simulink library "downlink_labels_lib"  (Simulink 6.6)
libraries: Telemetry_Lib x4, simulink x1
settings Model: Creator=cbuttril  LastModifiedBy=cbuttril

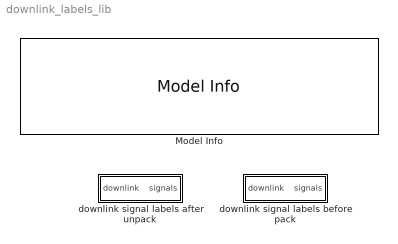
== system downlink_labels_lib ==
  Model Info : simulink/Model-Wide Utilities/Model Info  SystemSampleTime=-1  InitialBlockCM=None  BlockCM=None  Frame=on  DisplayStringWithTags=|  HorizontalTextAlignment=Center  LeftAlignmentValue=0.5  SourceBlockDiagram=downlink_labels_lib  TagMaxNumber=20
      | Developed using Matlab Release 2007a
      | 
      | SVN:%<ModelVersion>
      | Last modifed by %<LastModifiedBy> on %<LastModificationDate>
  downlink signal labels after unpack : Subsystem
  downlink signal labels before pack : Subsystem

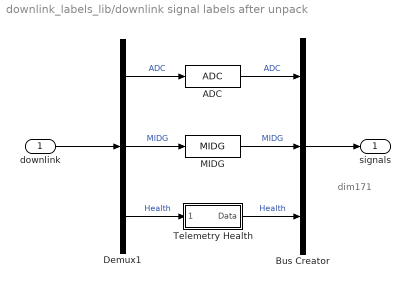
== system downlink_labels_lib/downlink signal labels after unpack ==
  note: dim171
  downlink : Inport
  ADC : Telemetry_Lib/ADC  SystemSampleTime=-1
  Bus Creator : BusCreator  Inputs=3
  Demux1 : Demux  Outputs=[62 99 10]
  MIDG : Telemetry_Lib/MIDG  SystemSampleTime=-1
  Telemetry Health : Subsystem
  signals : Outport  PortDimensions=171
  wires:
  Bus Creator/1 -> signals/1
  ADC/1 -> Bus Creator/1  "ADC"
  Demux1/1 -> ADC/1  "ADC"
  Telemetry Health/1(Data) -> Bus Creator/3  "Health"
  MIDG/1 -> Bus Creator/2  "MIDG"
  Demux1/3 -> Telemetry Health/1(Health)  "Health"
  Demux1/2 -> MIDG/1  "MIDG"
  downlink/1 -> Demux1/1

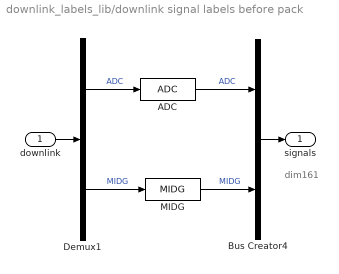
== system downlink_labels_lib/downlink signal labels before pack ==
  note: dim161
  downlink : Inport
  ADC : Telemetry_Lib/ADC  SystemSampleTime=-1
  Bus Creator4 : BusCreator  Inputs=2
  Demux1 : Demux  Outputs=[62 99]
  MIDG : Telemetry_Lib/MIDG  SystemSampleTime=-1
  signals : Outport  PortDimensions=161
  wires:
  ADC/1 -> Bus Creator4/1  "ADC"
  Demux1/1 -> ADC/1  "ADC"
  MIDG/1 -> Bus Creator4/2  "MIDG"
  Demux1/2 -> MIDG/1  "MIDG"
  downlink/1 -> Demux1/1
  Bus Creator4/1 -> signals/1

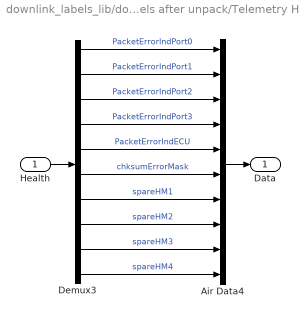
== system downlink_labels_lib/downlink signal labels after unpack/Telemetry Health ==
  Health : Inport
  Air Data4 : BusCreator  Inputs=10
  Demux3 : Demux  Outputs=10
  Data : Outport
  wires:
  Health/1 -> Demux3/1
  Air Data4/1 -> Data/1
  Demux3/10 -> Air Data4/10  "spareHM4"
  Demux3/9 -> Air Data4/9  "spareHM3"
  Demux3/8 -> Air Data4/8  "spareHM2"
  Demux3/7 -> Air Data4/7  "spareHM1"
  Demux3/6 -> Air Data4/6  "chksumErrorMask"
  Demux3/5 -> Air Data4/5  "PacketErrorIndECU"
  Demux3/4 -> Air Data4/4  "PacketErrorIndPort3"
  Demux3/3 -> Air Data4/3  "PacketErrorIndPort2"
  Demux3/2 -> Air Data4/2  "PacketErrorIndPort1"
  Demux3/1 -> Air Data4/1  "PacketErrorIndPort0"
